simulink model "Matrix1_PP"  (Simulink 9.0)
settings: Solver=FixedStepDiscrete  StartTime=0.0  StopTime=19800  FixedStep=200  RelTol=1e-3  EnableMultiTasking=on
model workspace (MAT data in the model file):
  already_pp = 1
  input_dataset = Simulink.SimulationData.Dataset
  input_dataset.any.Name = ''
  input_dataset.any.Version = 3
  input_dataset.any.Storage = Simulink.SimulationData.Storage.RamDatasetStorage
  input_dataset.any.Storage.any.Version = 2
  input_dataset.any.Storage.any.Elements{1} = Simulink.SimulationData.Signal
  input_dataset.any.Storage.any.Elements{1}.Version = 1
  input_dataset.any.Storage.any.Elements{1}.Values = timeseries
  input_dataset.any.Storage.any.Elements{1}.Values.Name = 'unnamed'
  input_dataset.any.Storage.any.Elements{1}.Values.DataInfo = tsdata.datametadata
  input_dataset.any.Storage.any.Elements{1}.Values.DataInfo.Interpolation = tsdata.interpolation
  input_dataset.any.Storage.any.Elements{1}.Values.DataInfo.Interpolation.Fhandle : function handle (value not decoded)
  input_dataset.any.Storage.any.Elements{1}.Values.DataInfo.Interpolation.Name = 'linear'
  input_dataset.any.Storage.any.Elements{1}.Values.TimeInfo = tsdata.timemetadata
  input_dataset.any.Storage.any.Elements{1}.Values.TimeInfo.Length = 100
  input_dataset.any.Storage.any.Elements{1}.Values.TimeInfo.DuplicateTimes = 0
  input_dataset.any.Storage.any.Elements{1}.Values.TimeInfo.Time_ = [0; 200; 400; 600; 800; 1000; 1200; 1400; 1600; 1800; 2000; 2200; 2400; 2600; 2800; 3000; 3200; 3400; 3600; 3800; 4000; 4200; 4400; 4600; 4800; 5000; 5200; 5400; 5600; 5800; 6000; 6200; 6400; 6600; 6800; 7000; 7200; 7400; 7600; 7800; 8000; 8200; 8400; 8600; 8800; 9000; 9200; 9400; 9600; 9800; 10000; 10200; 10400; 10600; 10800; 11000; 11200; 11400; 11600; 11800; 12000; 12200; 12400; 12600; 12800; 13000; 13200; 13400; 13600; 13800; 14000; 14200; 14400; 14600; 14800; 15000; 15200; 15400; 15600; 15800; 16000; 16200; 16400; 16600; 16800; 17000; 17200; 17400; 17600; 17800; 18000; 18200; 18400; 18600; 18800; 19000; 19200; 19400; 19600; 19800]
  input_dataset.any.Storage.any.Elements{1}.Values.TimeInfo.Initialized = 1
  input_dataset.any.Storage.any.Elements{1}.Values.QualityInfo = tsdata.qualmetadata
  input_dataset.any.Storage.any.Elements{1}.Values.Data_ = [86.5908781162; -72.8343704038; 186.948274969; 19.6953532797; -89.5637378539; 263.4009372; 225.565686896; 30.0938057391; 73.4850516007; 52.2268227189; -175.35462436; -119.252201832; -17.4459908894; -161.707103873; 206.585275617; -183.14142626; -164.446931417; -197.575171711; -163.40142131; -38.5807895377; -113.33862801; 254.027785262; -41.8755652022; -189.110207926; 242.928581208; 287.849027014; -36.6780161243; -233.328465936; -145.161182453; -54.7680923325; 56.9376444052; -142.672951331; 61.7058536292; 126.72946826; -166.95195959; -229.549409487; -121.994476069; -108.733018844; -45.4999441717; 4.71497079667; -248.690521746; -142.510659181; 180.608773662; -282.467833463; 257.312483687; 138.198517713; -6.83461571785; 47.1150366141; -157.629852137; -24.690703092; 277.853123572; 28.0834312434; 12.6814984824; -161.043367975; -6.6613536479; 74.4360529042; 107.481324519; -62.6908705988; -79.5380108733; 292.789201897; -277.356680256; 231.100804921; 247.972096584; 177.710324151; -240.772632807; -142.877289678; -98.7858960223; 107.836770826; -218.068117587; 132.736499149; -235.942883036; 92.2544092011; -3.49563801644; 167.431033939; 129.02224704; 242.232336334; 234.553502598; -99.5021683575; 119.247499401; -181.314103988; -281.675432217; 146.44455622; 0.0134613541205; -12.0467153124; 242.83334284; 65.9199890535; 70.5998337531; 215.665383388; 183.293654718; 46.0329093688; -190.246518351; -156.040793659; 231.907159846; -282.795508522; -6.05916689267; -199.243712591; 287.208389785; 127.616683007; 0.282974492906; -17.3469752748]
  input_dataset.any.Storage.any.Elements{1}.Name = 'E'
settings Model: SuppressorTable=22 serialization::archive 11 0 6 0 0 0 0 0  Creator=scaife  LastModifiedBy=hbourbou  ExtModeAutoUpdateStatusClock=off
settings DataIOCC: ExternalInput=input_dataset  LimitDataPoints=on  LoadExternalInput=on  SaveFormat=Dataset  SignalLoggingSaveFormat=ModelDataLogs  SaveState=on  SignalLoggingName=sigsOut
settings DebuggingCC: AlgebraicLoopMsg=error  SaveWithParameterizedLinksMsg=none  SignalResolutionControl=TryResolveAllWithWarning  MultiTaskDSMMsg=warning  MultiTaskCondExecSysMsg=none  StrictBusMsg=None
settings HardwareCC: TargetUnknown=on
settings SFSimCC: SimParseCustomCode=off
settings GRTTargetCC: GeneratePreprocessorConditionals=Disable all  CombineOutputUpdateFcns=off  GRTInterface=on  ExtMode=on

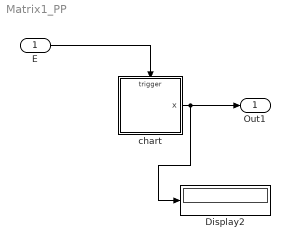
== system Matrix1_PP ==
  E : Inport
  Display2 : Display
  chart : Stateflow chart  TreatAsAtomicUnit=on
  Out1 : Outport
  wires:
  E/1 -> chart/Trigger
  chart/1(x) -> Out1/1, Display2/1

== stateflow chart chart ==
  state A/
    en:
    i = 3;
    x(1) = x(2,i) + 1;
  state B/
    en:x(2) = x(2,2) + 1;
  state C/
    en:x(3) = x(3) + 1;
  (default) -> A
  A -> B : E
  C -> A : E
  B -> C : E
  data: x output int32 size=[2 3] [0..100] =int32([1 2 3; 4 5 6]); i local double
  events: E input RISING_EDGE_EVENT
